simulink model "Gorev4"  (R2019a)
settings: Solver=VariableStepAuto  StartTime=0.0  StopTime=500  RelTol=1e-3
settings Model: Creator=handeyildirim  LastModifiedBy=handeyildirim

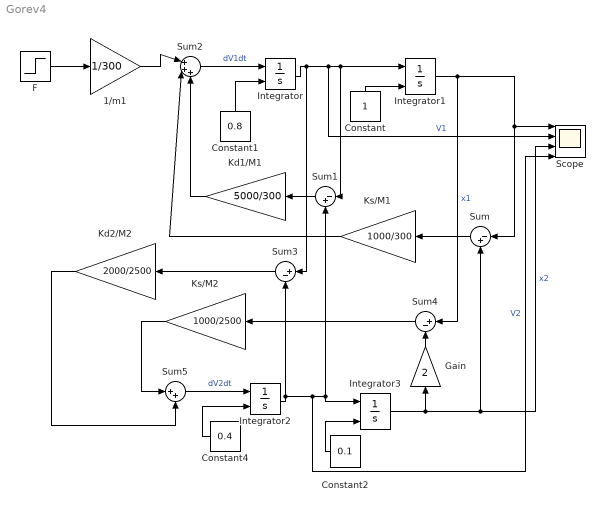
== system Gorev4 ==
  1/m1 : Gain  Gain=1/300
  Constant : Constant
  Constant1 : Constant  Value=0.8
  Constant2 : Constant  Value=0.1
  Constant4 : Constant  Value=0.4
  F : Step  Before=1000  After=1000  SampleTime=0
  Gain : Gain  Gain=2
  Integrator{,1..3} (4 alike) : Integrator  InitialConditionSource=external
  Kd1/M1 : Gain  Gain=5000/300
  Kd2/M2 : Gain  Gain=2000/2500
  Ks/M1 : Gain  Gain=1000/300
  Ks/M2 : Gain  Gain=1000/2500
  Scope : Scope  NumInputPorts=4
  Sum : Sum  Inputs=|-+
  Sum1 : Sum  Inputs=|-+
  Sum2 : Sum  Inputs=|+++
  Sum3 : Sum  Inputs=|+-
  Sum4 : Sum  Inputs=|+-
  Sum5 : Sum  Inputs=|++
  wires:
  Sum2/1 -> Integrator/1  "dV1dt"
  Integrator/1 -> Sum3/1, Scope/2, Sum1/1, Integrator1/1  "V1"
  Integrator3/1 -> Gain/1, Sum/2, Scope/3  "x2"
  Sum5/1 -> Integrator2/1  "dV2dt"
  Integrator2/1 -> Scope/4, Sum1/2, Integrator3/1, Sum3/2  "V2"
  Integrator1/1 -> Sum4/1, Sum/1, Scope/1  "x1"
  Sum/1 -> Ks/M1/1
  Sum1/1 -> Kd1/M1/1
  Kd1/M1/1 -> Sum2/3
  Ks/M1/1 -> Sum2/2
  1/m1/1 -> Sum2/1
  F/1 -> 1/m1/1
  Sum4/1 -> Ks/M2/1
  Gain/1 -> Sum4/2
  Sum3/1 -> Kd2/M2/1
  Kd2/M2/1 -> Sum5/2
  Ks/M2/1 -> Sum5/1
  Constant/1 -> Integrator1/2
  Constant1/1 -> Integrator/2
  Constant2/1 -> Integrator3/2
  Constant4/1 -> Integrator2/2
